simulink model "kre_ekf_validation"  (R2026a)
settings: Solver=FixedStepDiscrete  StopTime=0.2  FixedStep=5e-5
settings Model: Creator=hzldx  LastModifiedBy=hzldx

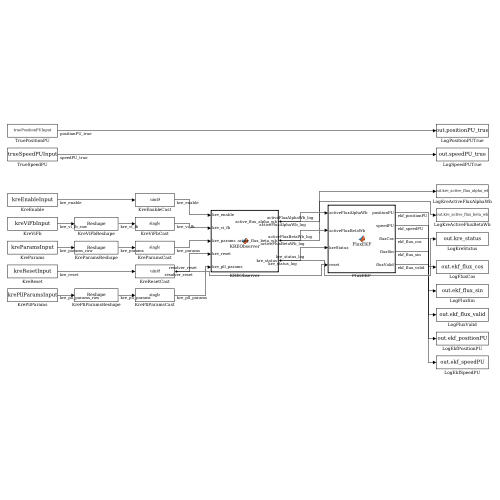
[thumbnail: Simulink's stored preview of the top-level diagram]
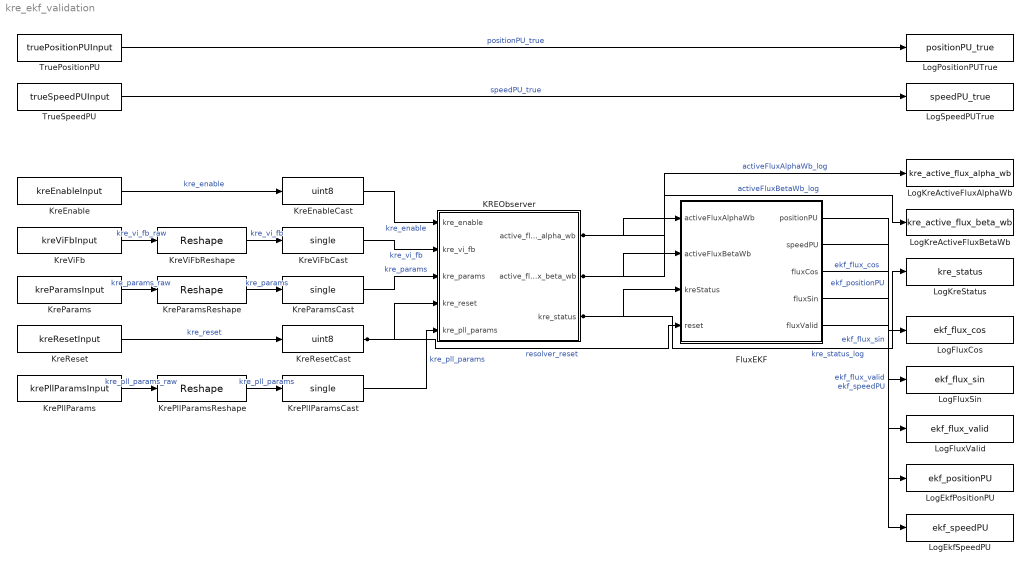
== system kre_ekf_validation ==
  FluxEKF : MATLAB Function  TreatAsAtomicUnit=on
  KREObserver : MATLAB Function  TreatAsAtomicUnit=on
  KreEnable : FromWorkspace  VariableName=kreEnableInput  Interpolate=off  OutputAfterFinalValue=Holding final value
  KreEnableCast : DataTypeConversion  OutDataTypeStr=uint8  SaturateOnIntegerOverflow=off  RndMeth=Floor
  KreParams : FromWorkspace  VariableName=kreParamsInput  Interpolate=off  OutputAfterFinalValue=Holding final value
  KreParamsCast : DataTypeConversion  OutDataTypeStr=single  SaturateOnIntegerOverflow=off  RndMeth=Floor
  KreParamsReshape : Reshape  OutputDimensionality=Customize  OutputDimensions=[14 1]
  KrePllParams : FromWorkspace  VariableName=krePllParamsInput  Interpolate=off  OutputAfterFinalValue=Holding final value
  KrePllParamsCast : DataTypeConversion  OutDataTypeStr=single  SaturateOnIntegerOverflow=off  RndMeth=Floor
  KrePllParamsReshape : Reshape  OutputDimensionality=Customize  OutputDimensions=[2 1]
  KreReset : FromWorkspace  VariableName=kreResetInput  Interpolate=off  OutputAfterFinalValue=Holding final value
  KreResetCast : DataTypeConversion  OutDataTypeStr=uint8  SaturateOnIntegerOverflow=off  RndMeth=Floor
  KreViFb : FromWorkspace  VariableName=kreViFbInput  Interpolate=off  OutputAfterFinalValue=Holding final value
  KreViFbCast : DataTypeConversion  OutDataTypeStr=single  SaturateOnIntegerOverflow=off  RndMeth=Floor
  KreViFbReshape : Reshape  OutputDimensionality=Customize  OutputDimensions=[4 1]
  LogEkfPositionPU : ToWorkspace  VariableName=ekf_positionPU  SaveFormat=Timeseries  SampleTime=-1
  LogEkfSpeedPU : ToWorkspace  VariableName=ekf_speedPU  SaveFormat=Timeseries  SampleTime=-1
  LogFluxCos : ToWorkspace  VariableName=ekf_flux_cos  SaveFormat=Timeseries  SampleTime=-1
  LogFluxSin : ToWorkspace  VariableName=ekf_flux_sin  SaveFormat=Timeseries  SampleTime=-1
  LogFluxValid : ToWorkspace  VariableName=ekf_flux_valid  SaveFormat=Timeseries  SampleTime=-1
  LogKreActiveFluxAlphaWb : ToWorkspace  VariableName=kre_active_flux_alpha_wb  SaveFormat=Timeseries  SampleTime=-1
  LogKreActiveFluxBetaWb : ToWorkspace  VariableName=kre_active_flux_beta_wb  SaveFormat=Timeseries  SampleTime=-1
  LogKreStatus : ToWorkspace  VariableName=kre_status  SaveFormat=Timeseries  SampleTime=-1
  LogPositionPUTrue : ToWorkspace  VariableName=positionPU_true  SaveFormat=Timeseries  SampleTime=-1
  LogSpeedPUTrue : ToWorkspace  VariableName=speedPU_true  SaveFormat=Timeseries  SampleTime=-1
  TruePositionPU : FromWorkspace  VariableName=truePositionPUInput  Interpolate=off  OutputAfterFinalValue=Holding final value
  TrueSpeedPU : FromWorkspace  VariableName=trueSpeedPUInput  Interpolate=off  OutputAfterFinalValue=Holding final value
  wires:
  TruePositionPU/1 -> LogPositionPUTrue/1  "positionPU_true"
  TrueSpeedPU/1 -> LogSpeedPUTrue/1  "speedPU_true"
  KreEnable/1 -> KreEnableCast/1  "kre_enable"
  KreViFb/1 -> KreViFbReshape/1  "kre_vi_fb_raw"
  KreViFbReshape/1 -> KreViFbCast/1  "kre_vi_fb"
  KreParams/1 -> KreParamsReshape/1  "kre_params_raw"
  KreParamsReshape/1 -> KreParamsCast/1  "kre_params"
  KreReset/1 -> KreResetCast/1  "kre_reset"
  KrePllParams/1 -> KrePllParamsReshape/1  "kre_pll_params_raw"
  KrePllParamsReshape/1 -> KrePllParamsCast/1  "kre_pll_params"
  KreEnableCast/1 -> KREObserver/1(kre_enable)  "kre_enable"
  KreViFbCast/1 -> KREObserver/2(kre_vi_fb)  "kre_vi_fb"
  KreParamsCast/1 -> KREObserver/3(kre_params)  "kre_params"
  KreResetCast/1 -> KREObserver/4(kre_reset), FluxEKF/4(reset)  "resolver_reset"
  KrePllParamsCast/1 -> KREObserver/5(kre_pll_params)  "kre_pll_params"
  KREObserver/1(active_flux_alpha_wb) -> FluxEKF/1(activeFluxAlphaWb), LogKreActiveFluxAlphaWb/1  "activeFluxAlphaWb_log"
  KREObserver/2(active_flux_beta_wb) -> FluxEKF/2(activeFluxBetaWb), LogKreActiveFluxBetaWb/1  "activeFluxBetaWb_log"
  KREObserver/3(kre_status) -> FluxEKF/3(kreStatus), LogKreStatus/1  "kre_status_log"
  FluxEKF/1(positionPU) -> LogEkfPositionPU/1  "ekf_positionPU"
  FluxEKF/2(speedPU) -> LogEkfSpeedPU/1  "ekf_speedPU"
  FluxEKF/3(fluxCos) -> LogFluxCos/1  "ekf_flux_cos"
  FluxEKF/4(fluxSin) -> LogFluxSin/1  "ekf_flux_sin"
  FluxEKF/5(fluxValid) -> LogFluxValid/1  "ekf_flux_valid"

== matlab function kre_ekf_validation/FluxEKF ==
  data: activeFluxAlphaWb input; positionPU output; activeFluxBetaWb input; kreStatus input; reset input; speedPU output; fluxCos output; fluxSin output; fluxValid output; resolver_ekf_config parameter
function [positionPU, speedPU, fluxCos, fluxSin, fluxValid] = ...
    FluxEKF(activeFluxAlphaWb, activeFluxBetaWb, kreStatus, reset, resolver_ekf_config)
%#codegen
persistent state initialized positionHold speedHold
if isempty(state)
    state = zeros(3, 1);
    initialized = false;
    positionHold = 0;
    speedHold = 0;
end
fluxCos = 0;
fluxSin = 0;
fluxValid = uint8(0);
if reset ~= 0
    state = zeros(3, 1);
    initialized = false;
    positionHold = 0;
    speedHold = 0;
end
if kreStatus == uint8(1)
    fluxAlpha = double(activeFluxAlphaWb);
    fluxBeta = double(activeFluxBetaWb);
    fluxMagnitude = sqrt(fluxAlpha * fluxAlpha + fluxBeta * fluxBeta);
    if isfinite(fluxMagnitude) && fluxMagnitude > 0
        fluxCos = fluxAlpha / fluxMagnitude;
        fluxSin = fluxBeta / fluxMagnitude;
        [state, positionHold, speedHold] = resolver_ekf_step( ...
            state, fluxCos, fluxSin, ~initialized, resolver_ekf_config);
        initialized = true;
        fluxValid = uint8(1);
    end
end
positionPU = positionHold;
speedPU = speedHold;
end

== matlab function kre_ekf_validation/KREObserver ==
  data: kre_enable input; active_flux_alpha_wb output; kre_vi_fb input; kre_params input; kre_reset input; kre_pll_params input; active_flux_beta_wb output; kre_status output
function [active_flux_alpha_wb, active_flux_beta_wb, kre_status] = ...
    KREObserver(kre_enable, kre_vi_fb, kre_params, kre_reset, kre_pll_params)
%#codegen
persistent state
if isempty(state)
    state = zeros(18, 1, 'single');
end
[state, active_flux_alpha_wb, active_flux_beta_wb, kre_status] = ...
    kre_ekf_kre_step(state, kre_enable, kre_vi_fb, kre_params, ...
    kre_reset, kre_pll_params);
end
